simulink model "Median_Block_Testing"  (R2021a)
settings: Solver=VariableStepAuto  StartTime=0.0  StopTime=7.93555  RelTol=1e-3
undefined symbols (not defined in the file): lambda2
libraries: dspsigops x4, dspquant2 x4, dspstat3 x1
(part 2 of 2)

== system Median_Block_Testing/Threshold_Estimator/Median2/Data_Sorter8 ==
  Signal1 : Inport  OutDataTypeStr=fixdt(1,16,12)  SampleTime=0.000022675736
  Signal2 : Inport  Port=2  OutDataTypeStr=fixdt(1,16,12)  SampleTime=0.000022675736
  Data_Sorter_Switch : Switch  OutDataTypeStr=fixdt(1,16,12)
  Data_Sorter_Switch1 : Switch  Threshold=1  OutDataTypeStr=fixdt(1,16,12)
  Delay1 : Delay  DelayLength=1  SampleTime=0.000022675736
  Delay2 : Delay  DelayLength=1  SampleTime=0.000022675736
  Relational Operator2 : RelationalOperator  Operator=<  OutDataTypeStr=fixdt(1,16,12)  RndMeth=Simplest
  High_Data : Outport  OutDataTypeStr=fixdt(1,16,12)  SampleTime=0.000022675736  VectorParamsAs1DForOutWhenUnconnected=off
  Low_Data : Outport  Port=2  OutDataTypeStr=fixdt(1,16,12)  SampleTime=0.000022675736  VectorParamsAs1DForOutWhenUnconnected=off
  wires:
  Signal1/1 -> Data_Sorter_Switch/3, Data_Sorter_Switch/1, Relational Operator2/1
  Relational Operator2/1 -> Data_Sorter_Switch1/2, Data_Sorter_Switch/2
  Signal2/1 -> Data_Sorter_Switch1/1, Data_Sorter_Switch1/3, Relational Operator2/2
  Data_Sorter_Switch1/1 -> Delay2/1
  Delay2/1 -> Low_Data/1
  Data_Sorter_Switch/1 -> Delay1/1
  Delay1/1 -> High_Data/1

== system Median_Block_Testing/Threshold_Estimator/Median2/Data_Sorter9 ==
  Signal1 : Inport  OutDataTypeStr=fixdt(1,16,12)  SampleTime=0.000022675736
  Signal2 : Inport  Port=2  OutDataTypeStr=fixdt(1,16,12)  SampleTime=0.000022675736
  Data_Sorter_Switch : Switch  OutDataTypeStr=fixdt(1,16,12)
  Data_Sorter_Switch1 : Switch  Threshold=1  OutDataTypeStr=fixdt(1,16,12)
  Delay1 : Delay  DelayLength=1  SampleTime=0.000022675736
  Delay2 : Delay  DelayLength=1  SampleTime=0.000022675736
  Relational Operator2 : RelationalOperator  Operator=<  OutDataTypeStr=fixdt(1,16,12)  RndMeth=Simplest
  High_Data : Outport  OutDataTypeStr=fixdt(1,16,12)  SampleTime=0.000022675736  VectorParamsAs1DForOutWhenUnconnected=off
  Low_Data : Outport  Port=2  OutDataTypeStr=fixdt(1,16,12)  SampleTime=0.000022675736  VectorParamsAs1DForOutWhenUnconnected=off
  wires:
  Signal1/1 -> Data_Sorter_Switch/3, Data_Sorter_Switch/1, Relational Operator2/1
  Relational Operator2/1 -> Data_Sorter_Switch1/2, Data_Sorter_Switch/2
  Signal2/1 -> Data_Sorter_Switch1/1, Data_Sorter_Switch1/3, Relational Operator2/2
  Data_Sorter_Switch1/1 -> Delay2/1
  Delay2/1 -> Low_Data/1
  Data_Sorter_Switch/1 -> Delay1/1
  Delay1/1 -> High_Data/1
